simulink model "mdlref_basic"  (Simulink 6.0)
settings: Solver=FixedStepDiscrete  SolverMode=SingleTasking  StartTime=0.0  StopTime=10.0  FixedStep=0.1  RelTol=1e-3
settings Model: Creator=The MathWorks Inc.  LastModifiedBy=batserve  ExtModeAutoUpdateStatusClock=off  ProdHWDeviceType=Specified
settings DataIOCC: SaveFormat=StructureWithTime  SignalLoggingName=logsOut
settings OptimizationCC: InlineParams=on
settings DebuggingCC: CheckExecutionContextPreStartOutputMsg=on  CheckExecutionContextRuntimeOutputMsg=on  SignalResolutionControl=UseLocalSettings  SolverPrmCheckMsg=none
settings HardwareCC: ProdHWDeviceType=Specified  TargetHWDeviceType=32-bit Generic  ProdEqTarget=off
settings ModelReferenceCC: UpdateModelReferenceTargets=IfOutOfDate  CheckModelReferenceTargetMessage=none
settings RTWCC: GenerateReport=on  ProcessScript=grt_make_rtw_hook  LaunchReport=on

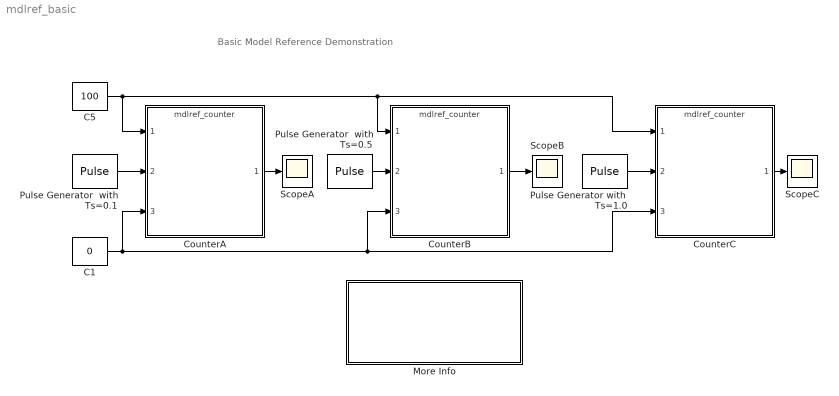
== system mdlref_basic ==
  note: Basic Model Reference Demonstration
  C1 : Constant  Value=0
  C5 : Constant  Value=100
  CounterA : ModelReference  ModelName=mdlref_counter  ModelReferenceVersion=1.64  CopyOfModelName=mdlref_counter
  CounterB : ModelReference  ModelName=mdlref_counter  ModelReferenceVersion=1.64  CopyOfModelName=mdlref_counter
  CounterC : ModelReference  ModelName=mdlref_counter  ModelReferenceVersion=1.64  CopyOfModelName=mdlref_counter
  More Info : Subsystem  PropExecContextAcrossSSBoundary=on
      settings: OpenFcn=mdlref_basicscript
      mask Display: disp('Double click here \nfor a step-by-step\ntutorial on this model')
  Pulse Generator  with Ts=0.1 : DiscretePulseGenerator  SampleTime=0.1  VectorParams1D=off
  Pulse Generator  with Ts=0.5 : DiscretePulseGenerator  SampleTime=0.5
  Pulse Generator with  Ts=1.0 : DiscretePulseGenerator  SampleTime=1.0
  ScopeA : Scope
      settings: TimeRange=10  YMin=0  YMax=100  SaveName=ScopeDataA
  ScopeB : Scope
      settings: TimeRange=10  YMin=0  YMax=25  SaveName=ScopeDataB
  ScopeC : Scope
      settings: TimeRange=10  YMin=0  YMax=15  SaveName=ScopeDataC
  wires:
  CounterB/1 -> ScopeB/1
  CounterA/1 -> ScopeA/1
  CounterC/1 -> ScopeC/1
  Pulse Generator  with Ts=0.1/1 -> CounterA/2
  Pulse Generator  with Ts=0.5/1 -> CounterB/2
  Pulse Generator with  Ts=1.0/1 -> CounterC/2
  C1/1 -> CounterA/3, CounterB/3, CounterC/3
  C5/1 -> CounterA/1, CounterB/1, CounterC/1

== system mdlref_basic/More Info ==
  note: Bus Block Demonstration
  note: This demonstration shows how signals may be grouped and ungrouped while
      | retaining their names.  In this demonstration, 5 signals are created and labelled
      | appropriately.  These signals are then mux'd together to create a bus of signals.
      | This bus of signals is then fed into the Bus Selector block.  Inside of the Bus
      | Selector block, the Pulse and Chirp signals are chosen to be output from the
      | original signal bus.
      |
      | It is possible to place a nest signal buses and then still retrieve the original signal
      | with its label.
